simulink model "sensor_subsystems_static"  (R2024b)
settings: Solver=VariableStepAuto  StartTime=0.0  StopTime=10.0  RelTol=1e-3
settings Model: Creator=aakas  LastModifiedBy=aakas

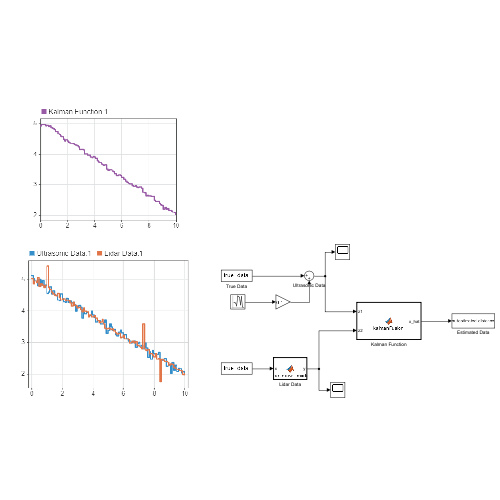
[thumbnail: Simulink's stored preview of the top-level diagram]
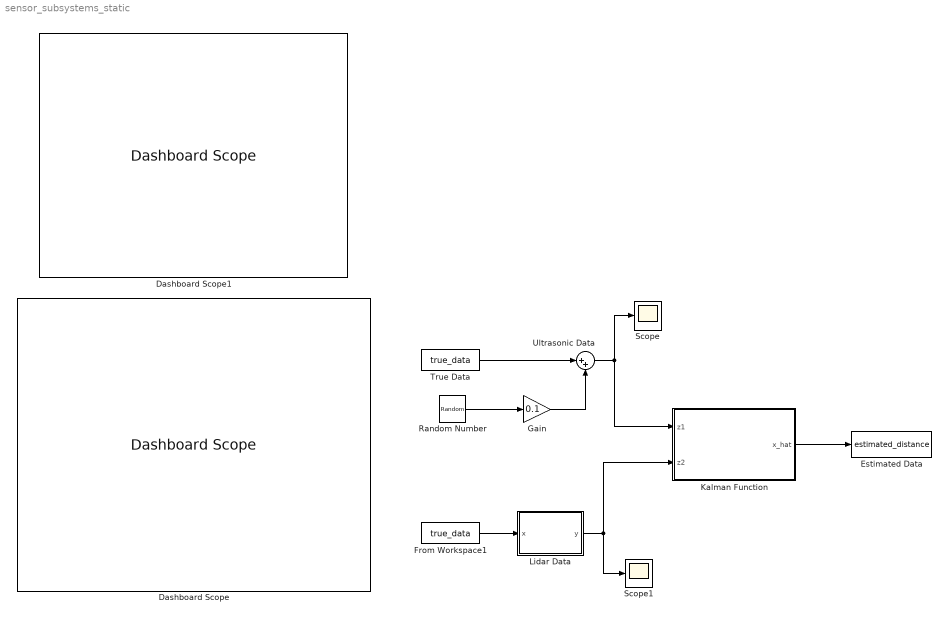
== system sensor_subsystems_static ==
  Dashboard Scope : DashboardScope
  Dashboard Scope1 : DashboardScope
  Estimated Data : ToWorkspace  VariableName=estimated_distance  SaveFormat=Timeseries  SampleTime=-1
  From Workspace1 : FromWorkspace  VariableName=true_data  SampleTime=0.1
  Gain : Gain  Gain=0.1
  Kalman Function : MATLAB Function  TreatAsAtomicUnit=on
  Lidar Data : MATLAB Function  TreatAsAtomicUnit=on
  Random Number : RandomNumber  SampleTime=0.1
  Scope : Scope
  Scope1 : Scope
  True Data : FromWorkspace  VariableName=true_data  SampleTime=0.1
  Ultrasonic Data : Sum  Inputs=|++
  wires:
  Random Number/1 -> Gain/1
  True Data/1 -> Ultrasonic Data/1
  Gain/1 -> Ultrasonic Data/2
  Ultrasonic Data/1 -> Scope/1, Kalman Function/1(z1)
  From Workspace1/1 -> Lidar Data/1(x)
  Lidar Data/1(y) -> Kalman Function/2(z2), Scope1/1
  Kalman Function/1(x_hat) -> Estimated Data/1

== matlab function sensor_subsystems_static/Lidar Data ==
  data: x input; y output
function y = lidar_noise_model(x)
% x: true distance
% y: noisy LiDAR reading

% Add small Gaussian noise
noise = 0.05 * randn();

% Random spike (5% chance)
if rand() < 0.05
    spike = 2 * (rand() - 0.5);  % Random spike between -1 and 1
else
    spike = 0;
end

y = x + noise + spike;

== matlab function sensor_subsystems_static/Kalman Function ==
  data: z1 input; x_hat output; z2 input
function x_hat = kalmanFusion(z1, z2)

%#codegen

persistent x P Q R1 R2 H I

if isempty(x)
    x = 0;                      % Initial estimate
    P = 1;                      % Initial error covariance
    Q = 0.01;                   % Process noise (decreasing this makes filter less responsive to change)
    R1 = 0.05;                  % LiDAR noise
    R2 = 0.2;                   % Ultrasonic noise (As we increase the noise here, the filter will start trusting LIdar more and viceversa
    H = 1;                      % Measurement model
    I = 1;                      % Identity matrix
end

% Measurement fusion (simple average or weighted)
z = (z1/R1 + z2/R2) / (1/R1 + 1/R2);
R = 1 / (1/R1 + 1/R2);  % Combined measurement noise

% Prediction
x_pred = x;
P_pred = P + Q;

% Update
K = P_pred * H / (H * P_pred * H + R);  % Kalman Gain
x = x_pred + K * (z - H * x_pred);
P = (I - K * H) * P_pred;

x_hat = x;
